simulink model "IandI_error_combinado"  (R2020b)
settings: Solver=ode45  StartTime=0.0  StopTime=100  FixedStep=0.0001  MaxStep=1e-3  RelTol=1e-8  EnableMultiTasking=on
StopFcn:
  | circulo2
undefined symbols (not defined in the file or in its folder): sigbuilder_block
settings Model: Creator=david  LastModifiedBy=dniet
settings DataIOCC: LimitDataPoints=on  SaveFormat=Array  ReturnWorkspaceOutputs=off
settings OptimizationCC: LifeSpan=inf
settings DebuggingCC: SolverPrmCheckMsg=warning  SFUnexpectedBacktrackingDiag=warning  SFNoUnconditionalDefaultTransitionDiag=warning  SFExecutionAtInitializationDiag=none  ArithmeticOperatorsInVariantConditions=warning
settings HardwareCC: ProdBitPerPointer=32  ProdBitPerSizeT=32  ProdBitPerPtrDiffT=32  ProdLargestAtomicFloat=None  ProdIntDivRoundTo=Undefined  ProdEndianess=Unspecified  ProdWordSize=32  ProdHWDeviceType=32-bit Generic
settings ModelReferenceCC: PropagateSignalLabelsOutOfModel=off
settings SFSimCC: SimUseLocalCustomCode=off  CustomCodeUndefinedFunction=UseInterfaceOnly
settings RTWCC: RTWUseLocalCustomCode=off
settings CodeAppCC: StateflowObjectComments=on
settings GRTTargetCC: TargetLangStandard=C89/C90 (ANSI)
settings ConfigComp: CovMetricSettings=dw  CovSaveCumulativeToWorkspaceVar=on  CovSaveSingleToWorkspaceVar=on  CovExternalEMLEnable=off  CovSFcnEnable=off

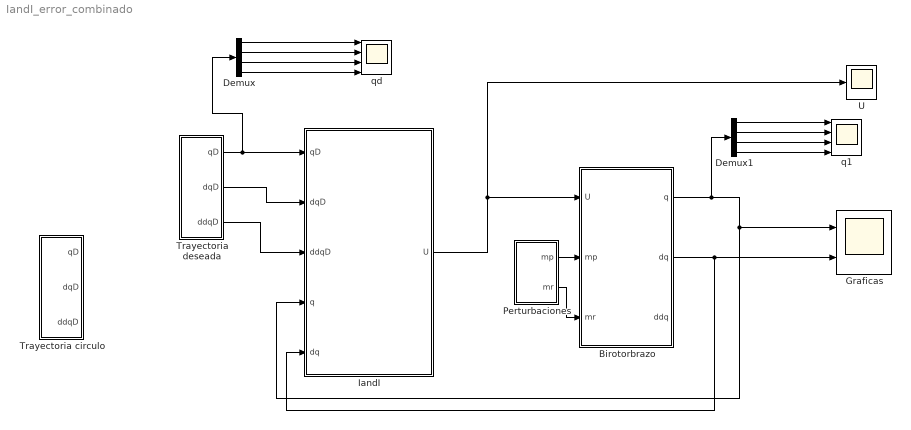
== system IandI_error_combinado ==
  Birotorbrazo : Subsystem
  Demux : Demux
  Demux1 : Demux
  Graficas : Scope  NumInputPorts=2
  IandI : MATLAB Function  TreatAsAtomicUnit=on
  Perturbaciones : Subsystem
  Trayectoria circulo : Subsystem
  Trayectoria deseada : Subsystem
  U : Scope
  q1 : Scope  NumInputPorts=4
  qd : Scope  NumInputPorts=4
  wires:
  Birotorbrazo/2(dq) -> IandI/5(dq), Graficas/2
  Demux/1 -> qd/1
  Demux/2 -> qd/2
  Birotorbrazo/1(q) -> Demux1/1, IandI/4(q), Graficas/1
  Demux1/3 -> q1/3
  Demux1/4 -> q1/4
  Demux/3 -> qd/3
  Demux/4 -> qd/4
  Trayectoria deseada/3(ddqD) -> IandI/3(ddqD)
  Trayectoria deseada/1(qD) -> IandI/1(qD), Demux/1
  Demux1/1 -> q1/1
  Demux1/2 -> q1/2
  Trayectoria deseada/2(dqD) -> IandI/2(dqD)
  Perturbaciones/1(mp) -> Birotorbrazo/2(mp)
  Perturbaciones/2(mr) -> Birotorbrazo/3(mr)
  IandI/1(U) -> Birotorbrazo/1(U), U/1

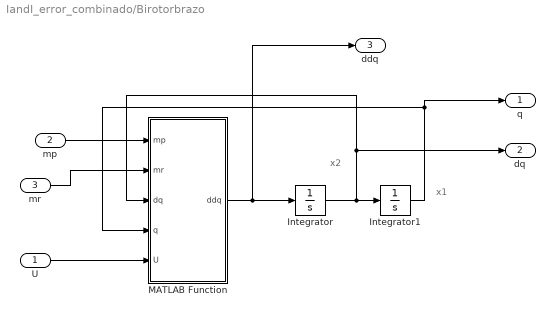
== system IandI_error_combinado/Birotorbrazo ==
  note: x2
  note: x1
  U : Inport
  mp : Inport  Port=2
  mr : Inport  Port=3
  Integrator : Integrator  InitialCondition=[0.001;0.001;0.001;0.001]
  Integrator1 : Integrator  InitialCondition=[0.01;0.01;pi/6-0.4;pi/6-0.3]
  MATLAB Function : MATLAB Function  TreatAsAtomicUnit=on
  q : Outport
  dq : Outport  Port=2
  ddq : Outport  Port=3
  wires:
  Integrator1/1 -> q/1, MATLAB Function/4(q)
  Integrator/1 -> MATLAB Function/3(dq), dq/1, Integrator1/1
  MATLAB Function/1(ddq) -> ddq/1, Integrator/1
  U/1 -> MATLAB Function/5(U)
  mr/1 -> MATLAB Function/2(mr)
  mp/1 -> MATLAB Function/1(mp)

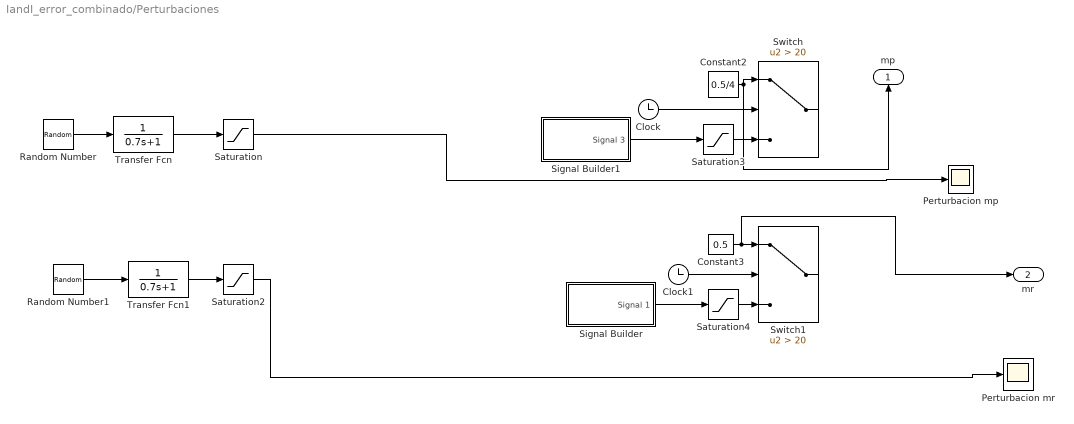
== system IandI_error_combinado/Perturbaciones ==
  Clock : Clock
  Clock1 : Clock
  Constant2 : Constant  Value=0.5/4
  Constant3 : Constant  Value=0.5
  Perturbacion mp : Scope
  Perturbacion mr : Scope
  Random Number : RandomNumber  Mean=0.5/4  Variance=(0.25)^2  SampleTime=0.1
  Random Number1 : RandomNumber  Mean=0.5  Variance=(0.5)^2  SampleTime=0.1
  Saturation : Saturate  UpperLimit=3  LowerLimit=0.05
  Saturation2 : Saturate  UpperLimit=3  LowerLimit=0.05
  Saturation3 : Saturate  UpperLimit=3  LowerLimit=0.01
  Saturation4 : Saturate  UpperLimit=3  LowerLimit=0.01
  Signal Builder : Subsystem  Tag=STV Subsys  LoadFcn=sigbuilder_block('load');  StartFcn=sigbuilder_block('start');  StopFcn=sigbuilder_block('stop');  ClipboardFcn=sigbuilder_block('clipboard');  mask(Sigbuilder block){tuvar=[0:10]}
      mask help: Simulink:masks:SigbuilderBlock_MD
      mask init:
      | if ~strcmp(get_param(bdroot(gcbh),'SimulationStatus'),'stopped') tuvar = sigbuilder_block('maskInit'); end
      settings: CopyFcn=sigbuilder_block('copy');  DeleteFcn=sigbuilder_block('delete');  ModelCloseFcn=sigbuilder_block('modelClose');  PreSaveFcn=sigbuilder_block('preSave');  PauseFcn=sigbuilder_block('pause');  ContinueFcn=sigbuilder_block('continue');  NameChangeFcn=sigbuilder_block('namechange');  OpenFcn=sigbuilder_block('open',[437.6 199.2 550.4 400 ]);  CloseFcn=sigbuilder_block('close');
      mask Display: plot(0, 0, 100, 100,[2, 2, 32, 32, 2], [68, 8, 8, 68, 68],[32, 2], [38, 38], [32, 19, 2],[53, 60, 44], [32, 17, 17, 2],[16, 16, 31, 31]);txt = getActiveGroup(gcbh);text(2, 100, txt,'verticalAlignment', 'top');
  Signal Builder1 : Subsystem  Tag=STV Subsys  LoadFcn=sigbuilder_block('load');  StartFcn=sigbuilder_block('start');  StopFcn=sigbuilder_block('stop');  ClipboardFcn=sigbuilder_block('clipboard');  mask(Sigbuilder block){tuvar=[0:10]}
      mask help: Simulink:masks:SigbuilderBlock_MD
      mask init:
      | if ~strcmp(get_param(bdroot(gcbh),'SimulationStatus'),'stopped') tuvar = sigbuilder_block('maskInit'); end
      settings: CopyFcn=sigbuilder_block('copy');  DeleteFcn=sigbuilder_block('delete');  ModelCloseFcn=sigbuilder_block('modelClose');  PreSaveFcn=sigbuilder_block('preSave');  PauseFcn=sigbuilder_block('pause');  ContinueFcn=sigbuilder_block('continue');  NameChangeFcn=sigbuilder_block('namechange');  OpenFcn=sigbuilder_block('open',[437.6 199.2 550.4 400 ]);  CloseFcn=sigbuilder_block('close');
      mask Display: plot(0, 0, 100, 100,[2, 2, 32, 32, 2], [68, 8, 8, 68, 68],[32, 2], [38, 38], [32, 19, 2],[53, 60, 44], [32, 17, 17, 2],[16, 16, 31, 31]);txt = getActiveGroup(gcbh);text(2, 100, txt,'verticalAlignment', 'top');
  Switch : Switch  Criteria=u2 > Threshold  Threshold=20
  Switch1 : Switch  Criteria=u2 > Threshold  Threshold=20
  Transfer Fcn : TransferFcn  Denominator=[0.7 1]
  Transfer Fcn1 : TransferFcn  Denominator=[0.7 1]
  mp : Outport
  mr : Outport  Port=2
  wires:
  Constant2/1 -> Switch/1, mp/1
  Saturation3/1 -> Switch/3
  Saturation4/1 -> Switch1/3
  Clock/1 -> Switch/2
  Constant3/1 -> mr/1, Switch1/1
  Clock1/1 -> Switch1/2
  Signal Builder/1(Signal 1) -> Saturation4/1
  Signal Builder1/1(Signal 3) -> Saturation3/1
  Random Number/1 -> Transfer Fcn/1
  Random Number1/1 -> Transfer Fcn1/1
  Transfer Fcn/1 -> Saturation/1
  Transfer Fcn1/1 -> Saturation2/1
  Saturation/1 -> Perturbacion mp/1
  Saturation2/1 -> Perturbacion mr/1

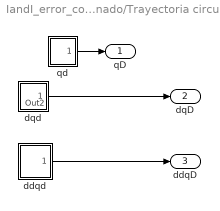
== system IandI_error_combinado/Trayectoria circulo ==
  ddqd : Subsystem
  dqd : Subsystem
      settings: PortSchema="{\"entries\":[{\"content\":{\"sides\":[{\"content\":{\"connectorIds\":[]},\"type\":\"ConnectorPlacement.EquallySpacedRectSide\",\"uuid\":\"acdd0822-6fcd-4af4-8f17-01735313a60e\"},{\"content\":{\"connectorIds\":[\"Out1\"],\"side\":\"RIGHT\"},\"type\":\"ConnectorPlacement.EquallySpacedRectSide\",\"uuid\":\"612510e7-c5e9-4dae-b30c-07af35f65a20\"},{\"content\":{\"connectorIds\":[],\"side\":\"TOP\"},\"type\":\"ConnectorPlacement.EquallySpacedRectSide\",\"uuid\":\"af5c6190-6ff2-4983-b61e-e34e07bda4fd\"},{\"content\":{\"connectorIds\":[\"Out2\"],\"side\":\"BOTTOM\"},\"type\":\"ConnectorPlacement.EquallySpacedRectSide\",\"uuid\":\"dee39b03-aed6-4b1e-80a4-9bb61a7b874d\"},{\"content\":{\"connectorIds\":[],\"side\":\"HIDDEN\"},\"type\":\"ConnectorPlacement.EquallySpacedRectSide\",\"uuid\":\"bb9a4ee1-278f-42c4-9d20-485988fb9c26\"}]},\"type\":\"ConnectorPlacement.EquallySpacedConnector\",\"uuid\":\"1c24b2b1-dbdf-424b-9692-27251213bdd0\"}],\"packageUris\":[\"http://schema.mathworks.com/mf0/Connector/R2020b\"],\"version\":\"1.0\"}"
  qd : Subsystem
  qD : Outport
  dqD : Outport  Port=2
  ddqD : Outport  Port=3
  wires:
  qd/1(qd) -> qD/1
  dqd/1(dqd) -> dqD/1
  ddqd/1(ddqD) -> ddqD/1

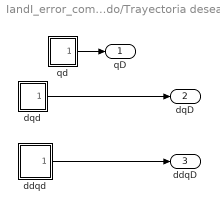
== system IandI_error_combinado/Trayectoria deseada ==
  ddqd : Subsystem
  dqd : Subsystem
  qd : Subsystem
  qD : Outport
  dqD : Outport  Port=2
  ddqD : Outport  Port=3
  wires:
  qd/1(qd) -> qD/1
  dqd/1(dqd) -> dqD/1
  ddqd/1(ddqD) -> ddqD/1

== system IandI_error_combinado/Perturbaciones/Signal Builder ==
  Demux : Demux  Tag=STV Demux  Outputs=1
      settings: DisplayOption=none
  FromWs : FromWorkspace  Tag=STV FromWs  VariableName=tuvar
      SigBuilderData=|
      | common.afterFinalStr = 'Extrapolate'
      | common.sampleTime = 0
      | dataSet.timeRange = [0 20]
      | dataSet.name = 'Group 1'
      | sbobj.Groups.Name = 'Group 1'
      | sbobj.Groups.Signals.Name = 'Signal 1'
      | sbobj.Groups.Signals.XData = [0 0.5 1 1.5 2 2.5 3 3.5 4 4.5 5 5.5 6 6.5 7 7.5 8 8.5 9 9.5 10 10.5 11 11.5 12 12.5 13 13.5 14 14.5 15 15.5 16 16.5 17 17.5 18 18.5 19 19.5 20]
      | sbobj.Groups.Signals.YData = [0.442869805681 0.333726697686 0.304158738967 0.268719668867 0.393288578137 0.0994728528234 0.692845884526 0.604012020291 0.495994429671 0.493045782794 0.340367283087 0.703737056426 0.473356504098 0.357093967243 0.770277153685 0.455045788789 0.382194193856 0.441249280453 0.330414751272 0.275974339751 1.00519993842 0.831099518577 0.561507031848 0.24857632813 0.326906393889 0.464693177154 0.658283212326 0.233599115737 0.065 0.210180541432 0.566702166613 0.578270720887 0.590335883786 0.473943069371 0.536737819172 0.404769396676 0.672404322311 0.227661105826 0.591005911289 0.330258124013 0.433022612207]
      | sbobj.Groups.TimeRange = [0 20]
  Signal 1 : Outport  Tag=STV Outport
  wires:
  FromWs/1 -> Demux/1
  Demux/1 -> Signal 1/1

== system IandI_error_combinado/Perturbaciones/Signal Builder1 ==
  Demux : Demux  Tag=STV Demux  Outputs=1
      settings: DisplayOption=none
  FromWs : FromWorkspace  Tag=STV FromWs  VariableName=tuvar
      SigBuilderData=|
      | common.afterFinalStr = 'Extrapolate'
      | common.sampleTime = 0
      | dataSet.timeRange = [0 20]
      | dataSet.name = 'Group 1'
      | sbobj.Groups.Name = 'Group 1'
      | sbobj.Groups.Signals.Name = 'Signal 3'
      | sbobj.Groups.Signals.XData = [0 0.5 1 1.5 2 2.5 3 3.5 4 4.5 5 5.5 6 6.5 7 7.5 8 8.5 9 9.5 10 10.5 11 11.5 12 12.5 13 13.5 14 14.5 15 15.5 16 16.5 17 17.5 18 18.5 19 19.5 20]
      | sbobj.Groups.Signals.YData = [0.135009283314 0.0705471070009 0.155352079465 0.0649673437866 0.173996532117 0.19893631236 0.296188778298 0.105587646424 0.015 0.0410411252663 0.2604594328 0.0177844711616 0.221095386974 0.13740498 0.268669662272 0.055 0.105230177403 0.14 0.415800803073 0.207521889423 0.262897197792 0.0191819742013 0.0781384418899 0.097753059075 0.234842461789 0.0972128067212 0.195154145816 0.02 0.0896150002226 0.0426413474843 0.01 0.175797465091 0.153198406367 0.128347988224 0.035 0.237749227834 0.16001794106 0.0950933969667 0.127288979275 0.0988004565034 0.03]
      | sbobj.Groups.TimeRange = [0 20]
  Signal 3 : Outport  Tag=STV Outport
  wires:
  FromWs/1 -> Demux/1
  Demux/1 -> Signal 3/1

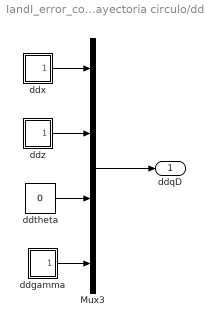
== system IandI_error_combinado/Trayectoria circulo/ddqd ==
  Mux3 : Mux
  ddgamma : Subsystem
  ddtheta : Constant  Value=0
  ddx : Subsystem
  ddz : Subsystem
  ddqD : Outport
  wires:
  ddz/1(ddz) -> Mux3/2
  Mux3/1 -> ddqD/1
  ddx/1(ddx) -> Mux3/1
  ddtheta/1 -> Mux3/3
  ddgamma/1(ddgamma) -> Mux3/4

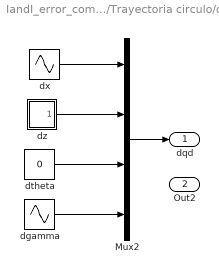
== system IandI_error_combinado/Trayectoria circulo/dqd ==
  Mux2 : Mux
  dgamma : Sin  Amplitude=pi/12  Frequency=1/2  Phase=pi/2  SampleTime=0
  dtheta : Constant  Value=0
  dx : Sin  Amplitude=2  Frequency=1/2  Phase=pi/2  SampleTime=0
  dz : Subsystem
  dqd : Outport
  Out2 : Outport  Port=2
  wires:
  dz/1(dz) -> Mux2/2
  Mux2/1 -> dqd/1
  dx/1 -> Mux2/1
  dtheta/1 -> Mux2/3
  dgamma/1 -> Mux2/4

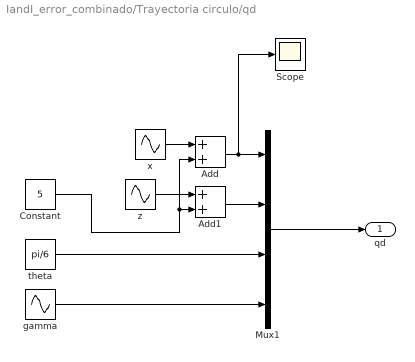
== system IandI_error_combinado/Trayectoria circulo/qd ==
  Add : Sum
  Add1 : Sum
  Constant : Constant  Value=5
  Mux1 : Mux
  Scope : Scope
  gamma : Sin  Amplitude=pi/6  Frequency=1/2  SampleTime=0
  theta : Constant  Value=pi/6
  x : Sin  Amplitude=4  Frequency=1/2  SampleTime=0
  z : Sin  Amplitude=4  Frequency=1/2  Phase=pi/2  SampleTime=0
  qd : Outport
  wires:
  Mux1/1 -> qd/1
  theta/1 -> Mux1/3
  Add/1 -> Scope/1, Mux1/1
  Add1/1 -> Mux1/2
  z/1 -> Add1/1
  x/1 -> Add/1
  Constant/1 -> Add1/2, Add/2
  gamma/1 -> Mux1/4

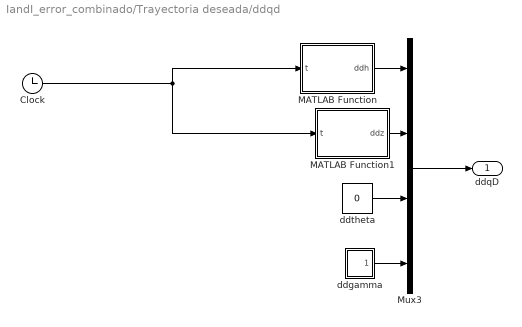
== system IandI_error_combinado/Trayectoria deseada/ddqd ==
  Clock : Clock
  MATLAB Function : MATLAB Function  TreatAsAtomicUnit=on
  MATLAB Function1 : MATLAB Function  TreatAsAtomicUnit=on
  Mux3 : Mux
  ddgamma : Subsystem
  ddtheta : Constant  Value=0
  ddqD : Outport
  wires:
  Mux3/1 -> ddqD/1
  ddtheta/1 -> Mux3/3
  ddgamma/1(ddgamma) -> Mux3/4
  MATLAB Function/1(ddh) -> Mux3/1
  MATLAB Function1/1(ddz) -> Mux3/2
  Clock/1 -> MATLAB Function1/1(t), MATLAB Function/1(t)

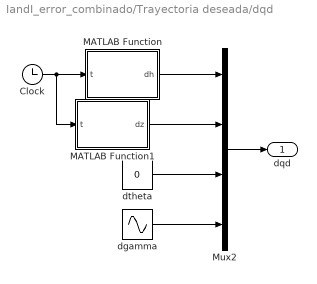
== system IandI_error_combinado/Trayectoria deseada/dqd ==
  Clock : Clock
  MATLAB Function : MATLAB Function  TreatAsAtomicUnit=on
  MATLAB Function1 : MATLAB Function  TreatAsAtomicUnit=on
  Mux2 : Mux
  dgamma : Sin  Amplitude=pi/12  Frequency=1/2  Phase=pi/2  SampleTime=0
  dtheta : Constant  Value=0
  dqd : Outport
  wires:
  MATLAB Function1/1(dz) -> Mux2/2
  Mux2/1 -> dqd/1
  MATLAB Function/1(dh) -> Mux2/1
  dtheta/1 -> Mux2/3
  dgamma/1 -> Mux2/4
  Clock/1 -> MATLAB Function1/1(t), MATLAB Function/1(t)

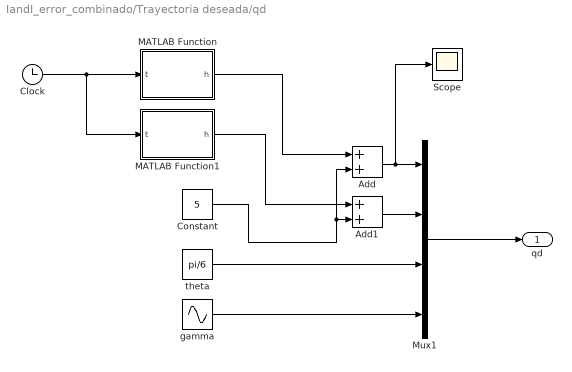
== system IandI_error_combinado/Trayectoria deseada/qd ==
  Add : Sum
  Add1 : Sum
  Clock : Clock
  Constant : Constant  Value=5
  MATLAB Function : MATLAB Function  TreatAsAtomicUnit=on
  MATLAB Function1 : MATLAB Function  TreatAsAtomicUnit=on
  Mux1 : Mux
  Scope : Scope
  gamma : Sin  Amplitude=pi/6  Frequency=1/2  SampleTime=0
  theta : Constant  Value=pi/6
  qd : Outport
  wires:
  Mux1/1 -> qd/1
  theta/1 -> Mux1/3
  Add/1 -> Scope/1, Mux1/1
  Add1/1 -> Mux1/2
  Constant/1 -> Add1/2, Add/2
  gamma/1 -> Mux1/4
  Clock/1 -> MATLAB Function1/1(t), MATLAB Function/1(t)
  MATLAB Function/1(h) -> Add/1
  MATLAB Function1/1(h) -> Add1/1

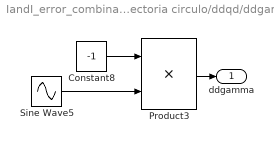
== system IandI_error_combinado/Trayectoria circulo/ddqd/ddgamma ==
  Constant8 : Constant  Value=-1
  Product3 : Product
  Sine Wave5 : Sin  Amplitude=pi/24  Frequency=1/2  SampleTime=0
  ddgamma : Outport
  wires:
  Sine Wave5/1 -> Product3/2
  Constant8/1 -> Product3/1
  Product3/1 -> ddgamma/1

== system IandI_error_combinado/Trayectoria circulo/ddqd/ddx ==
  Constant8 : Constant  Value=-1
  Product3 : Product
  Sine Wave5 : Sin  Frequency=1/2  SampleTime=0
  ddx : Outport
  wires:
  Sine Wave5/1 -> Product3/2
  Constant8/1 -> Product3/1
  Product3/1 -> ddx/1

== system IandI_error_combinado/Trayectoria circulo/ddqd/ddz ==
  Constant2 : Constant  Value=-1
  Product : Product
  cos : Sin  Frequency=1/2  Phase=pi/2  SampleTime=0
  ddz : Outport
  wires:
  Product/1 -> ddz/1
  Constant2/1 -> Product/1
  cos/1 -> Product/2

== system IandI_error_combinado/Trayectoria circulo/dqd/dz ==
  Constant2 : Constant  Value=-1
  Product : Product
  cos : Sin  Amplitude=2  Frequency=1/2  SampleTime=0
  dz : Outport
  wires:
  Product/1 -> dz/1
  Constant2/1 -> Product/1
  cos/1 -> Product/2

== system IandI_error_combinado/Trayectoria deseada/ddqd/ddgamma ==
  Constant8 : Constant  Value=-1
  Product3 : Product
  Sine Wave5 : Sin  Amplitude=pi/24  Frequency=1/2  SampleTime=0
  ddgamma : Outport
  wires:
  Sine Wave5/1 -> Product3/2
  Constant8/1 -> Product3/1
  Product3/1 -> ddgamma/1

== matlab function IandI_error_combinado/Birotorbrazo/MATLAB Function ==
  data: mp input; mr input; ddq output; dq input; q input; U input
function ddq = fcn(mp, mr,dq,q,U)
%#codegen
lp = 0.35;
g = 9.81;
%mr = 0.5;
Ir = 0.177;
%mp = 0.5/4;

vphi = q(3);
%eta = q(4);
dvphi = dq(3);
deta = dq(4);

Mq = [(mr+mp),0,mp*lp*cos(vphi),0;0,(mr+mp),mp*lp*sin(vphi),0;mp*lp*cos(vphi),mp*lp*sin(vphi),mp*(lp^2),0;0,0,0,mp*(lp^2)+Ir];
Cq = [0,0,-dvphi*mp*lp*sin(vphi),0;0,0,dvphi*mp*lp*cos(vphi),0;0,0,0,0;0,0,0,0];
gq = [0;(mr+mp)*g;mp*lp*sin(vphi)*g;0];

ddq = Mq\(-Cq*dq-gq+U);

== matlab function IandI_error_combinado/IandI ==
  data: qD input; dqD input; U output; ddqD input; q input; dq input
function U = fcn(qD,dqD,ddqD,q,dq)
%#codegen
lp = 0.35;
g = 9.81;
mr = 0.5;
Ir = 0.177;
mp=0.5/4;

%A=10000;
%B= -20000/exp(1);

vphi = q(3);
%eta = q(4);
dvphi = dq(3);
%deta = dq(4);

Gan2= 200/(100*exp(1));
Gan=100/100;
ks=eye(4)*Gan2;
KGan2=eye(4)*Gan;

ddqr=ddqD-KGan2*(dq-dqD);
dqr= dqD-KGan2*(q-qD);
s=dq-dqD+KGan2*(q-qD);
%k2=eye(4)*B; %B= -((2 Exp^(-s* t))/t^2)
%k1=eye(4)*A; %A=-((Exp^(-s *t) (-2 Exp+Exp^(s* t) s^2 t^2))/t^2)

%qt=q-qD;

Mq = [(mr+mp),0,mp*lp*cos(vphi),0;0,(mr+mp),mp*lp*sin(vphi),0;mp*lp*cos(vphi),mp*lp*sin(vphi),mp*(lp^2),0;0,0,0,mp*(lp^2)+Ir];
Cq = [0,0,-dvphi*mp*lp*sin(vphi),0;0,0,dvphi*mp*lp*cos(vphi),0;0,0,0,0;0,0,0,0];
gq = [0;(mr+mp)*g;mp*lp*sin(vphi)*g;0];
U = Mq*ddqr + Cq*dqr+gq-ks*s;

== matlab function IandI_error_combinado/Trayectoria deseada/qd/MATLAB Function ==
  data: t input; h output
function h = fcn(t)

h = 5*cos(5*t*pi/100)*cos(t*pi/100);

== matlab function IandI_error_combinado/Trayectoria deseada/qd/MATLAB Function1 ==
  data: t input; h output
function h = fcn(t)

h = 5*cos(5*t*pi/100)*sin(t*pi/100);

== matlab function IandI_error_combinado/Trayectoria deseada/dqd/MATLAB Function ==
  data: t input; dh output
function dh = fcn(t)
dh=-(1/20)*pi*(2*sin(pi*t/25) + 3*sin(3 *pi* t/50));

== matlab function IandI_error_combinado/Trayectoria deseada/dqd/MATLAB Function1 ==
  data: t input; dz output
function dz = fcn(t)
dz=(1/20)*pi*(-2*cos(pi*t/25) + 3*cos(3 *pi* t/50));

== matlab function IandI_error_combinado/Trayectoria deseada/ddqd/MATLAB Function ==
  data: t input; ddh output
function ddh = fcn(t)
ddh=-((pi^2 *(4* cos((pi*t)/25) + 9*cos((3 *pi* t)/50)))/1000);

== matlab function IandI_error_combinado/Trayectoria deseada/ddqd/MATLAB Function1 ==
  data: t input; ddz output
function ddz = fcn(t)
ddz=((pi^2 *(4* sin((pi*t)/25) - 9*sin((3 *pi* t)/50)))/1000);
